simulink model "sphere"  (R2023b)
settings: Solver=ode4  StartTime=0  StopTime=100  FixedStep=0.01  MaxStep=0.01  RelTol=1e-3  EnableMultiTasking=on
values from neighbouring files (symbols this model uses):
  simu = simulationClass()    [wecSimInputFile.m]    (also in wecSimInputFile_FreeDecay.m)
  waves = waveClass('regular')    [wecSimInputFile.m]    (also in wecSimInputFile_FreeDecay.m = waveClass('noWaveCIC'))
undefined symbols (not defined in the file or in its folder): body, pto, X, Y, Z
libraries: nesl_utility x24, sm_lib x17, WECSim_Lib_Body_Elements x6, vrlib x1, WECSim_Lib_Frames x1, WECSim_Lib_PTOs x1
(part 4 of 4)

== matlab function sphere/Float/Hydrodynamic Body/Yaw Kinematic Transforms/With B2B/Yaw Kinematic Transforms ==
  data: yaw input; dispLoc output; dispGlobal input; velGlobal input; accGlobal input; velLoc output; accLoc output; numBody parameter
function [dispLoc, velLoc, accLoc] = kinYawTransformB2B(yaw, dispGlobal, velGlobal, accGlobal, numBody)

[dispLoc, velLoc, accLoc] = kinYawTransformB2B(yaw, dispGlobal, velGlobal, accGlobal, numBody);

end

== matlab function sphere/Float/Hydrodynamic Body/Morison Element and Viscous Damping Force Calculation/Morison Element Variant Subsystem/Morison Element On/Regular Wave Morison Force/MATLAB Function ==
  data: z input; f output; r input; Vel input; Accel input; Disp input; Area input; Cd input; Vol input; Ca input; Time input; rho input; waveDir input; waterDepth input; k input; w input; A input; rampTime input; g input; currentSpeed input; currentDirection input; currentDepth input; currentOption input; simuMorison input
function f = regWaveMorison(z,r,Vel,Accel,Disp,Area,Cd,Vol,Ca,Time,rho,waveDir,waterDepth,k,w,A,rampTime,g,currentSpeed,currentDirection,currentDepth,currentOption,simuMorison)

f = regWaveMorison(z,r,Vel,Accel,Disp,Area,Cd,Vol,Ca,Time,rho,waveDir,waterDepth,k,w,A,rampTime,g,currentSpeed,currentDirection,currentDepth,currentOption,simuMorison);

end

== matlab function sphere/Float/Hydrodynamic Body/Wave Diffraction and Excitation Force Calculation/Linear Wave Excitation Force Variant Subsystem/Irregular Wave NonLinearYaw/MATLAB Function1 ==
  data: disp input; dispPhase output; enable input; frequency input; wavenumber input; direction input
function dispPhase  = calcDispPhase(disp, enable, frequency, wavenumber, direction)
% initialize
dispPhase = zeros(length(frequency),length(direction));
% execute
dispPhase = calcDispPhase(disp, enable, direction, frequency, wavenumber);

end

== matlab function sphere/Float/Hydrodynamic Body/Wave Diffraction and Excitation Force Calculation/Linear Wave Excitation Force Variant Subsystem/Irregular Wave Full Direction/MATLAB Function ==
  data: pYaw input; nBins input; A input; w input; nW input; dofGRD input; dirGRD input; wGRD input; qDofGRD input; qWGRD input; fEHRE input; fEHIM input; Fext output; relYawLast output; fEHMD input; phaseRand input; dw input; time input; spreadBins input; dirBins input; Disp input; intThresh input; prevYaw input; prevCoeffMD input; prevCoeffRE input; prevCoeffIM input; coeffsLastMD output; coeffsLastRE output; coeffsLastIM output
function [Fext, relYawLast, coeffsLastMD,coeffsLastRE,coeffsLastIM] = irregExcFullDirF(pYaw, nBins, A,w, nW, dofGRD,dirGRD,wGRD,qDofGRD,qWGRD,fEHRE,fEHIM, fEHMD, phaseRand,dw,time,spreadBins, dirBins, Disp, intThresh, prevYaw, prevCoeffMD, prevCoeffRE, prevCoeffIM)

[Fext,relYawLast,coeffsLastMD,coeffsLastRE,coeffsLastIM] = irregExcFullDirF(pYaw,nBins,A,w,nW,dofGRD,dirGRD,wGRD,qDofGRD,qWGRD,fEHRE,fEHIM, fEHMD, phaseRand,dw,time,spreadBins, dirBins, Disp, intThresh, prevYaw, prevCoeffMD, prevCoeffRE, prevCoeffIM);

end

== matlab function sphere/Float/Hydrodynamic Body/Wave Diffraction and Excitation Force Calculation/Linear Wave Excitation Force Variant Subsystem/Irregular Wave Full Direction/MATLAB Function1 ==
  data: disp input; dispPhase output; enable input; frequency input; wavenumber input; nBins input
function dispPhase  = calcDispPhase(disp, enable, frequency, wavenumber, nBins)
% initialize
dispPhase = zeros(length(frequency),length(nBins));
% execute
dispPhase = calcDispPhase(disp, enable, nBins, frequency, wavenumber);

end

== matlab function sphere/Float/Hydrodynamic Body/Hydrostatic Restoring Force Calculation/Linear and Nonlinear Restoring Force Variant Subsystem/Nonlinear Hydrostatic Restoring Force/Restoring Forces ==
  data: x input; elv input; center input; f output; tnorm input; area input; rho input; g input; cg input; p output; mass input
function [f,p]  = nonLinearBuoyancy(x,elv,center,tnorm,area,rho,g,cg,mass)

[f,p]  = nonLinearBuoyancy(x,elv,center,tnorm,area,rho,g,cg,mass);

end

== matlab function sphere/MATLAB Function ==
  data: zDisp input; body1_hydroForceIndex output
function body1_hydroForceIndex = calcIndex(zDisp)

body1_hydroForceIndex = calcIndex(zDisp);

end

== matlab function sphere/Float/Hydrodynamic Body/Wave Diffraction and Excitation Force Calculation/Linear Wave Excitation Force Variant Subsystem/Irregular Wave NonLinearYaw/MATLAB Function ==
  data: A input; w input; dofGRD input; dirGRD input; wGRD input; fEHRE input; fEHIM input; Fext output; fEHMD input; phaseRand input; dw input; time input; direction input; spread input; Disp input; intThresh input; prevYaw input; relYawLast output; prevCoeffMD input; prevCoeffRE input; prevCoeffIM input; coeffsLastMD output; coeffsLastRE output; coeffsLastIM output
function [Fext,relYawLast,coeffsLastMD,coeffsLastRE,coeffsLastIM] = irregnLYaw(A,w,dofGRD,dirGRD,wGRD,fEHRE,fEHIM, fEHMD, phaseRand,dw,time,direction,spread, Disp, intThresh, prevYaw, prevCoeffMD, prevCoeffRE, prevCoeffIM)

%initialize outputs
Fext = zeros(1,6);
relYawLast=0;
coeffsLastMD=zeros(length(w),6);
coeffsLastRE=zeros(length(w),6);
coeffsLastIM=zeros(length(w),6);

[Fext,relYawLast,coeffsLastMD,coeffsLastRE,coeffsLastIM] = irregnLYaw(A,w,dofGRD,dirGRD,wGRD,fEHRE,fEHIM, fEHMD, phaseRand,dw,time,direction,spread, Disp, intThresh, prevYaw, prevCoeffMD, prevCoeffRE, prevCoeffIM);

end
